simulink library "libEngineThrustCalc"  (R2020b)
settings: Solver=VariableStepAuto  StartTime=0.0  StopTime=10.0  RelTol=1e-3
libraries: libEngineThrustLookUpTables x3
settings Model: Creator=caatay  LastModifiedBy=caatay

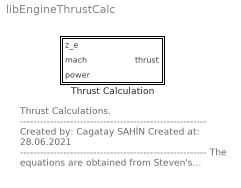
== system libEngineThrustCalc ==
  note: Thrust Calculations.
      | --------------------------------------------------------
      | Created by: Cagatay SAHİN
      | Created at: 28.06.2021
      | --------------------------------------------------------
      | The equations are obtained from
      | Steven's textbook.
      | The reference book can be found in
      | "references folder".
      | --------------------------------------------------------
      | for question:
      | cagataysahin44@gmail.com
  Thrust Calculation : Subsystem  mask(Engine Model - Thrust Calculation){}
      mask help: Aircraft's thrust calculation with using look-up thrust tables, atmospheric informations and state variables.
      mask Help:
      | This block is used for obtain thrust values with using atmospheric parameters and state information.
      | --------------------------------------------------------------------------------------------------------------------------------------------------
      | Input of the function:
      | 	pow: Actual Power (hP)
      | 	mach: Mach Number
      |                   z_e: Altitude (ft)
      | Output of the function:
      | 	T: Thrust (lbf)
      | --------------------------------------------------------------------------------------------------------------------------------------------------
      | All equations can be found in Steven's text book. Reference can be found in "literature" subfolder.
      | for question: "cagataysahin44@gmail.com"
      mask Display:
      | port_label('input',1,'z_{e}','texmode','on');
      | port_label('input',2,'mach','texmode','on');
      | port_label('input',3,'Pow','texmode','on');
      | 
      | port_label('output',1,'thrust','texmode','on');

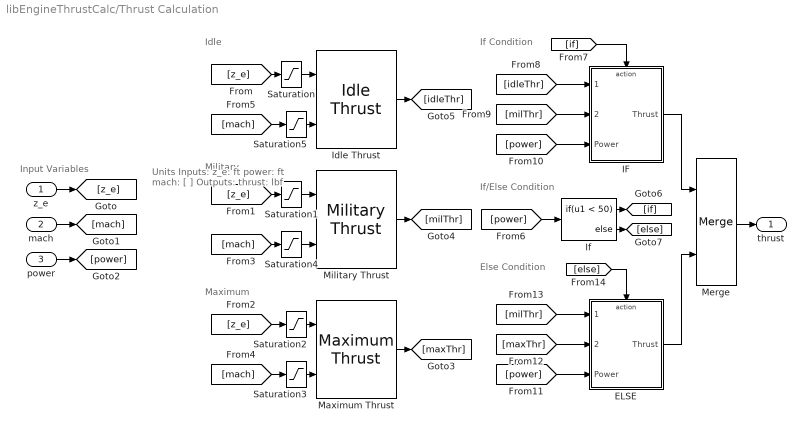
== system libEngineThrustCalc/Thrust Calculation ==
  note: Maximum
  note: Military
  note: Input Variables
  note: Units
      | Inputs:
      | z_e: ft
      | power: ft
      | mach: [ ]
      | Outputs:
      | thrust: lbf
  note: Idle
  note: If/Else Condition
  note: If Condition
  note: Else Condition
  z_e : Inport
  mach : Inport  Port=2
  power : Inport  Port=3
  ELSE : Subsystem  TreatAsAtomicUnit=on
  IF : Subsystem  TreatAsAtomicUnit=on
  Idle Thrust : libEngineThrustLookUpTables/Idle Thrust  data=data
  If : If  IfExpression=u1 < 50
  Maximum Thrust : libEngineThrustLookUpTables/Maximum Thrust  data=data
  Merge : Merge
  Military Thrust : libEngineThrustLookUpTables/Military Thrust  data=data
  Saturation : Saturate  UpperLimit=50000  LowerLimit=0
  Saturation1 : Saturate  UpperLimit=50000  LowerLimit=0
  Saturation2 : Saturate  UpperLimit=50000  LowerLimit=0
  Saturation3 : Saturate  UpperLimit=1  LowerLimit=0
  Saturation4 : Saturate  UpperLimit=1  LowerLimit=0
  Saturation5 : Saturate  UpperLimit=1  LowerLimit=0
  thrust : Outport  VectorParamsAs1DForOutWhenUnconnected=off
  wires:
  [maxThr] -> ELSE/2(Max Thrust)
  Merge/1 -> thrust/1
  ELSE/1(Thrust) -> Merge/2
  [power] -> ELSE/3(Power)
  [milThr] -> ELSE/1(Mil Thrust)
  [else] -> ELSE/Action
  IF/1(Thrust) -> Merge/1
  [power] -> IF/3(Power)
  [milThr] -> IF/2(Mil Thrust)
  [idleThr] -> IF/1(Idle Thrust)
  [if] -> IF/Action
  If/2 -> [else]
  If/1 -> [if]
  [power] -> If/1
  Idle Thrust/1 -> [idleThr]
  Military Thrust/1 -> [milThr]
  Maximum Thrust/1 -> [maxThr]
  power/1 -> [power]
  Saturation5/1 -> Idle Thrust/2
  [mach] -> Saturation5/1
  [mach] -> Saturation4/1
  Saturation4/1 -> Military Thrust/2
  Saturation3/1 -> Maximum Thrust/2
  [mach] -> Saturation3/1
  Saturation2/1 -> Maximum Thrust/1
  [z_e] -> Saturation2/1
  Saturation1/1 -> Military Thrust/1
  [z_e] -> Saturation1/1
  Saturation/1 -> Idle Thrust/1
  [z_e] -> Saturation/1
  z_e/1 -> [z_e]
  mach/1 -> [mach]

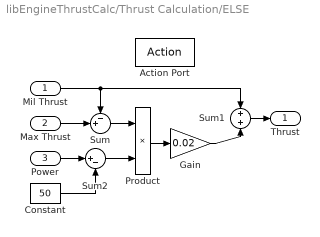
== system libEngineThrustCalc/Thrust Calculation/ELSE ==
  Mil Thrust : Inport
  Max Thrust : Inport  Port=2
  Power : Inport  Port=3
  Action Port : ActionPort
  Constant : Constant  Value=50
  Gain : Gain  Gain=0.02
  Product : Product
  Sum : Sum  Inputs=-+|
  Sum1 : Sum
  Sum2 : Sum  Inputs=|+-
  Thrust : Outport  VectorParamsAs1DForOutWhenUnconnected=off
  wires:
  Mil Thrust/1 -> Sum1/1, Sum/1
  Constant/1 -> Sum2/2
  Sum2/1 -> Product/2
  Product/1 -> Gain/1
  Sum/1 -> Product/1
  Sum1/1 -> Thrust/1
  Gain/1 -> Sum1/2
  Power/1 -> Sum2/1
  Max Thrust/1 -> Sum/2

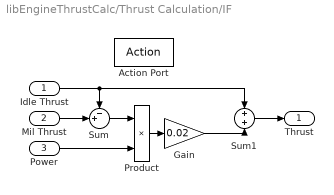
== system libEngineThrustCalc/Thrust Calculation/IF ==
  Idle Thrust : Inport
  Mil Thrust : Inport  Port=2
  Power : Inport  Port=3
  Action Port : ActionPort
  Gain : Gain  Gain=0.02
  Product : Product
  Sum : Sum  Inputs=-+|
  Sum1 : Sum
  Thrust : Outport  VectorParamsAs1DForOutWhenUnconnected=off
  wires:
  Gain/1 -> Sum1/2
  Sum1/1 -> Thrust/1
  Product/1 -> Gain/1
  Power/1 -> Product/2
  Sum/1 -> Product/1
  Mil Thrust/1 -> Sum/2
  Idle Thrust/1 -> Sum/1, Sum1/1
